simulink model "wawaw"  (R2026a)
settings: Solver=FixedStepAuto  StopTime=10  FixedStep=0.002

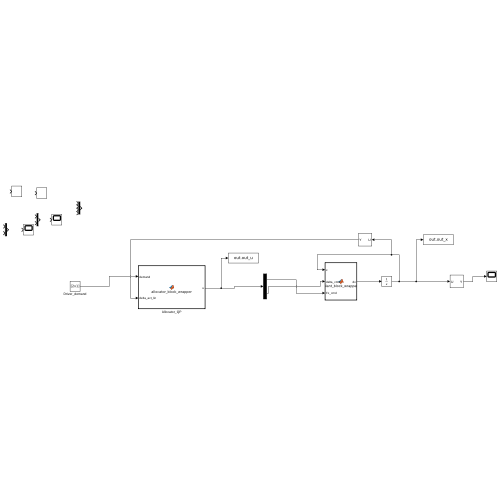
[thumbnail: Simulink's stored preview of the top-level diagram]
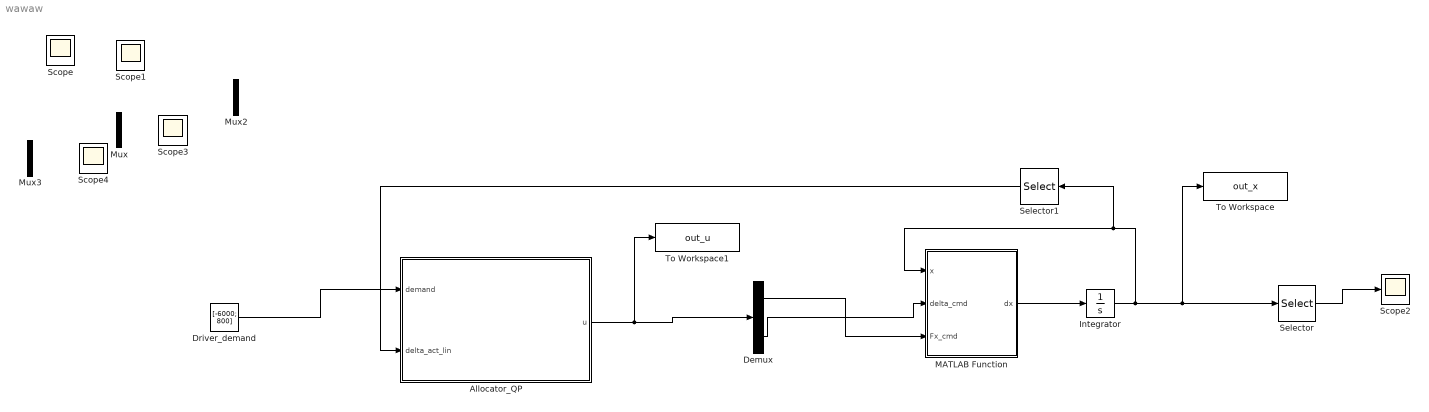
== system wawaw ==
  Allocator_QP : MATLAB Function  TreatAsAtomicUnit=on
  Demux : Demux  Outputs=[4 1]
  Driver_demand : Constant  Value=[-6000; 800]
  Integrator : Integrator  InitialCondition=[25;0;0;0;0;0;0;0;0;0;0]
  MATLAB Function : MATLAB Function  TreatAsAtomicUnit=on
  Mux : Mux  Inputs=2
  Mux2 : Mux
  Mux3 : Mux  Inputs=2
  Scope{,1..4} (5 alike) : Scope
      Scope settings: ActiveDisplayYMinimum=-26.913621383048014  ActiveDisplayYMaximum=31.992376142168563
      Scope1 settings: ActiveDisplayYMinimum=-0.048665724239335746  ActiveDisplayYMaximum=0.43799151815402182
      Scope2 settings: ActiveDisplayYMinimum=-3.1249999999999991  ActiveDisplayYMaximum=28.125  DataLoggingVariableName=ScopeData2
      Scope3 settings: ActiveDisplayYMinimum=-0.024673518179534129  ActiveDisplayYMaximum=0.22206166361580723  DataLoggingVariableName=ScopeData3
      Scope4 settings: ActiveDisplayYMinimum=-645.29307251823741  ActiveDisplayYMaximum=5807.6376526641379  DataLoggingVariableName=ScopeData4
  Selector : Selector  InputPortWidth=11  IndexOptions=Index vector (dialog)  Indices=[1 3 7]  OutputSizes=1
  Selector1 : Selector  InputPortWidth=11  IndexOptions=Index vector (dialog)  Indices=[7]  OutputSizes=1
  To Workspace : ToWorkspace  VariableName=out_x  SampleTime=-1
  To Workspace1 : ToWorkspace  VariableName=out_u  SampleTime=-1
  wires:
  MATLAB Function/1(dx) -> Integrator/1
  Selector/1 -> Scope2/1
  Driver_demand/1 -> Allocator_QP/1(demand)
  Allocator_QP/1(u) -> To Workspace1/1, Demux/1
  Demux/1 -> MATLAB Function/3(Fx_cmd)
  Demux/2 -> MATLAB Function/2(delta_cmd)
  Integrator/1 -> Selector1/1, MATLAB Function/1(x), To Workspace/1, Selector/1
  Selector1/1 -> Allocator_QP/2(delta_act_lin)

== matlab function wawaw/Allocator_QP ==
  data: demand input; u output; delta_act_lin input
function u = allocator_block_wrapper(demand, delta_act_lin)
coder.extrinsic('allocator');
u = zeros(5,1);
u = allocator(demand(:), delta_act_lin, []);
u = u(:);
end

== matlab function wawaw/MATLAB Function ==
  data: x input; dx output; delta_cmd input; Fx_cmd input
function dx = plant_block_wrapper(x, delta_cmd, Fx_cmd)
x = x(:);
Fx_cmd = Fx_cmd(:);
assert(numel(x) == 11);
assert(isequal(size(delta_cmd), [1 1]));
assert(numel(Fx_cmd) == 4);
dx = vehicle_derivatives_block(x, delta_cmd, Fx_cmd);
dx = dx(:);
assert(numel(dx) == 11);
end
